simulink model "ASM2d_Influentmodel"  (Simulink 7.0)
settings: Solver=ode45  StartTime=0.0  StopTime=728.0  RelTol=1e-6
values from neighbouring files (symbols this model uses):
  aHpercent = 75    [ASM2d_Influent_init.m]    (also in ASM3_Influent_init.m)
  CODpart_gperPEperd = 115.08    [ASM2d_Influent_init.m]    (also in ASM3_Influent_init.m)
  CODpart_HH_max = 20*CODpart_gperPEperd*PE    (= 184128)    [ASM2d_Influent_init.m]    (also in ASM3_Influent_init.m)
  CODpart_HH_min = 0.1    [ASM2d_Influent_init.m]    (also in ASM3_Influent_init.m)
  CODpart_HH_ns = 35000    [ASM2d_Influent_init.m]    (also in ASM3_Influent_init.m)
  CODpart_HH_nv = factor1*CODpart_gperPEperd*PE    (= 18412.8)    [ASM2d_Influent_init.m]    (also in ASM3_Influent_init.m)
  CODpart_HH_st = 1/24    (= 0.0416666666667)    [ASM2d_Influent_init.m]    (also in ASM3_Influent_init.m)
  CODpart_Ind_kgperd = 2301.80    (= 2301.8)    [ASM2d_Influent_init.m]    (also in ASM3_Influent_init.m)
  CODpart_Ind_max = 20*CODpart_Ind_kgperd    (= 46036)    [ASM2d_Influent_init.m]    (also in ASM3_Influent_init.m)
  CODpart_Ind_min = 0.1    [ASM2d_Influent_init.m]    (also in ASM3_Influent_init.m)
  CODpart_Ind_ns = 21000    [ASM2d_Influent_init.m]    (also in ASM3_Influent_init.m)
  CODpart_Ind_nv = factor2*CODpart_Ind_kgperd    (= 4603.6)    [ASM2d_Influent_init.m]    (also in ASM3_Influent_init.m)
  CODpart_Ind_st = 1/24    (= 0.0416666666667)    [ASM2d_Influent_init.m]    (also in ASM3_Influent_init.m)
  CODsol_gperPEperd = 19.31    [ASM2d_Influent_init.m]    (also in ASM3_Influent_init.m)
  CODsol_HH_max = 20*CODsol_gperPEperd*PE    (= 30896)    [ASM2d_Influent_init.m]    (also in ASM3_Influent_init.m)
  CODsol_HH_min = 0.1    [ASM2d_Influent_init.m]    (also in ASM3_Influent_init.m)
  CODsol_HH_ns = 25000    [ASM2d_Influent_init.m]    (also in ASM3_Influent_init.m)
  CODsol_HH_nv = factor1*2*CODsol_gperPEperd*PE    (= 6179.2)    [ASM2d_Influent_init.m]    (also in ASM3_Influent_init.m)
  CODsol_HH_st = 1/24    (= 0.0416666666667)    [ASM2d_Influent_init.m]    (also in ASM3_Influent_init.m)
  CODsol_Ind_kgperd = 386.24    [ASM2d_Influent_init.m]    (also in ASM3_Influent_init.m)
  CODsol_Ind_max = 20*CODsol_Ind_kgperd    (= 7724.8)    [ASM2d_Influent_init.m]    (also in ASM3_Influent_init.m)
  CODsol_Ind_min = 0.1    [ASM2d_Influent_init.m]    (also in ASM3_Influent_init.m)
  CODsol_Ind_ns = 11000    [ASM2d_Influent_init.m]    (also in ASM3_Influent_init.m)
  CODsol_Ind_nv = factor2*CODsol_Ind_kgperd    (= 772.48)    [ASM2d_Influent_init.m]    (also in ASM3_Influent_init.m)
  CODsol_Ind_st = 1/24    (= 0.0416666666667)    [ASM2d_Influent_init.m]    (also in ASM3_Influent_init.m)
  FFfraction = 0.25    [ASM2d_Influent_init.m]    (also in ASM3_Influent_init.m)
  HHnoiseswitch = 1    [ASM2d_Influent_init.m]    (also in ASM3_Influent_init.m)
  HHpolnoiseswitch = 1    [ASM2d_Influent_init.m]    (also in ASM3_Influent_init.m)
  HHpopswitch = 100    [ASM2d_Influent_init.m]    (also in ASM3_Influent_init.m)
  Indnoiseswitch = 1    [ASM2d_Influent_init.m]    (also in ASM3_Influent_init.m)
  Indpolnoiseswitch = 1    [ASM2d_Influent_init.m]    (also in ASM3_Influent_init.m)
  Indpopswitch = 100    [ASM2d_Influent_init.m]    (also in ASM3_Influent_init.m)
  InfAmp = 1200    [ASM2d_Influent_init.m]    (also in ASM3_Influent_init.m)
  InfBias = 7100    [ASM2d_Influent_init.m]    (also in ASM3_Influent_init.m)
  Infcst = 7100    [ASM2d_Influent_init.m]    (also in ASM3_Influent_init.m)
  InfFreq = 2*pi/364    (= 0.0172614980966)    [ASM2d_Influent_init.m]    (also in ASM3_Influent_init.m)
  InfPhase = -pi*15/24    (= -1.96349540849)    [ASM2d_Influent_init.m]    (also in ASM3_Influent_init.m)
  iSS_XB = 0.90    (= 0.9)    [ASM2d_Influent_init.m]
  iSS_XI = 0.75    [ASM2d_Influent_init.m]
  iSS_XMe = 1.00    (= 1)    [ASM2d_Influent_init.m]
  iSS_XPHA = 0.60    (= 0.6)    [ASM2d_Influent_init.m]
  iSS_XPP = 3.23    [ASM2d_Influent_init.m]
  iSS_XS = 0.75    [ASM2d_Influent_init.m]
  LLrain = 3.5    [ASM2d_Influent_init.m]    (also in ASM3_Influent_init.m)
  PE = 80    [ASM2d_Influent_init.m]    (also in ASM3_Influent_init.m)
  PO4_gperPEperd = (6.89*0.85)/4    (= 1.464125)    [ASM2d_Influent_init.m]
  PO4_HH_max = 20*PO4_gperPEperd*PE    (= 2342.6)    [ASM2d_Influent_init.m]
  PO4_HH_min = 0.1    [ASM2d_Influent_init.m]
  PO4_HH_ns = 55000    [ASM2d_Influent_init.m]
  PO4_HH_nv = factor1*2*PO4_gperPEperd*PE    (= 468.52)    [ASM2d_Influent_init.m]
  PO4_HH_st = 1/24    (= 0.0416666666667)    [ASM2d_Influent_init.m]
  PO4_Ind_kgperd = (61.25*0.85)/4    (= 13.015625)    [ASM2d_Influent_init.m]
  PO4_Ind_max = 20*PO4_Ind_kgperd    (= 260.3125)    [ASM2d_Influent_init.m]
  PO4_Ind_min = 0.1    [ASM2d_Influent_init.m]
  PO4_Ind_ns = 41000    [ASM2d_Influent_init.m]
  PO4_Ind_nv = factor2*PO4_Ind_kgperd    (= 26.03125)    [ASM2d_Influent_init.m]
  PO4_Ind_st = 1/24    (= 0.0416666666667)    [ASM2d_Influent_init.m]
  polnoiseswitch = 1    [ASM2d_Influent_init.m]    (also in ASM3_Influent_init.m)
  Q_HH_ns = 3857    [ASM2d_Influent_init.m]    (also in ASM3_Influent_init.m)
  Q_HH_nv = 4000    [ASM2d_Influent_init.m]    (also in ASM3_Influent_init.m)
  Q_HH_st = 1/24    (= 0.0416666666667)    [ASM2d_Influent_init.m]    (also in ASM3_Influent_init.m)
  Q_Ind_ns = 2000    [ASM2d_Influent_init.m]    (also in ASM3_Influent_init.m)
  Q_Ind_nv = 15000    [ASM2d_Influent_init.m]    (also in ASM3_Influent_init.m)
  Q_Ind_st = 1/24    (= 0.0416666666667)    [ASM2d_Influent_init.m]    (also in ASM3_Influent_init.m)
  Q_SCI_ns = 1000    [ASM2d_Influent_init.m]    (also in ASM3_Influent_init.m)
  Q_SCI_nv = 0.1*InfBias    (= 710)    [ASM2d_Influent_init.m]    (also in ASM3_Influent_init.m)
  Q_SCI_st = 1    [ASM2d_Influent_init.m]    (also in ASM3_Influent_init.m)
  QHHsatmax = QperPE*50    (= 7500)    [ASM2d_Influent_init.m]    (also in ASM3_Influent_init.m)
  QHHsatmin = 0.001    [ASM2d_Influent_init.m]    (also in ASM3_Influent_init.m)
  QInd_weekday = 2500    [ASM2d_Influent_init.m]    (also in ASM3_Influent_init.m)
  QIndsatmax = QInd_weekday*10    (= 25000)    [ASM2d_Influent_init.m]    (also in ASM3_Influent_init.m)
  QIndsatmin = 0.001    [ASM2d_Influent_init.m]    (also in ASM3_Influent_init.m)
  Qpermm = 1500    [ASM2d_Influent_init.m]    (also in ASM3_Influent_init.m)
  QperPE = 150    [ASM2d_Influent_init.m]    (also in ASM3_Influent_init.m)
  QSCIsatmax = 2*(InfBias+InfAmp)    (= 16600)    [ASM2d_Influent_init.m]    (also in ASM3_Influent_init.m)
  QSCIsatmin = 0.0    (= 0)    [ASM2d_Influent_init.m]    (also in ASM3_Influent_init.m)
  rain_nm = 1    [ASM2d_Influent_init.m]    (also in ASM3_Influent_init.m)
  rain_ns = 3000    [ASM2d_Influent_init.m]    (also in ASM3_Influent_init.m)
  rain_nv = 400    [ASM2d_Influent_init.m]    (also in ASM3_Influent_init.m)
  rain_st = 1/24    (= 0.0416666666667)    [ASM2d_Influent_init.m]    (also in ASM3_Influent_init.m)
  rainmax = 1000    [ASM2d_Influent_init.m]    (also in ASM3_Influent_init.m)
  rainmin = 0    [ASM2d_Influent_init.m]    (also in ASM3_Influent_init.m)
  rainpopswitch = 100    [ASM2d_Influent_init.m]    (also in ASM3_Influent_init.m)
  SA_max = 100*Sa_in    (= 2780)    [ASM2d_Influent_init.m]
  SA_min = 0.1    [ASM2d_Influent_init.m]
  SA_ns = 03122    (= 3122)    [ASM2d_Influent_init.m]
  SA_nv = factor3*(Sa_in)    (= 55.6)    [ASM2d_Influent_init.m]
  SA_st = 1/24    (= 0.0416666666667)    [ASM2d_Influent_init.m]
  SCInoiseswitch = 0    [ASM2d_Influent_init.m]    (also in ASM3_Influent_init.m)
  SCIpopswitch = 100    [ASM2d_Influent_init.m]    (also in ASM3_Influent_init.m)
  SF_max = 100*Sf_in    (= 4170)    [ASM2d_Influent_init.m]
  SF_min = 0.1    [ASM2d_Influent_init.m]
  SF_ns = 23122    [ASM2d_Influent_init.m]
  SF_nv = factor3*(Sf_in)    (= 83.4)    [ASM2d_Influent_init.m]
  SF_st = 1/24    (= 0.0416666666667)    [ASM2d_Influent_init.m]
  SI_max = 100*Si_in    (= 3000)    [ASM2d_Influent_init.m]    (also in ASM3_Influent_init.m)
  SI_min = 0.1    [ASM2d_Influent_init.m]    (also in ASM3_Influent_init.m)
  SI_ns = 13122    [ASM2d_Influent_init.m]    (also in ASM3_Influent_init.m)
  SI_nv = factor3*(Si_in)    (= 60)    [ASM2d_Influent_init.m]    (also in ASM3_Influent_init.m)
  SI_st = 1/24    (= 0.0416666666667)    [ASM2d_Influent_init.m]    (also in ASM3_Influent_init.m)
  SNH_gperPEperd = 6.89*0.85    (= 5.8565)    [ASM2d_Influent_init.m]    (also in ASM3_Influent_init.m)
  SNH_HH_max = 20*SNH_gperPEperd*PE    (= 9370.4)    [ASM2d_Influent_init.m]    (also in ASM3_Influent_init.m)
  SNH_HH_min = 0.1    [ASM2d_Influent_init.m]    (also in ASM3_Influent_init.m)
  SNH_HH_ns = 45000    [ASM2d_Influent_init.m]    (also in ASM3_Influent_init.m)
  SNH_HH_nv = factor1*2*SNH_gperPEperd*PE    (= 1874.08)    [ASM2d_Influent_init.m]    (also in ASM3_Influent_init.m)
  SNH_HH_st = 1/24    (= 0.0416666666667)    [ASM2d_Influent_init.m]    (also in ASM3_Influent_init.m)
  SNH_Ind_kgperd = 61.25*0.85    (= 52.0625)    [ASM2d_Influent_init.m]    (also in ASM3_Influent_init.m)
  SNH_Ind_max = 20*SNH_Ind_kgperd    (= 1041.25)    [ASM2d_Influent_init.m]    (also in ASM3_Influent_init.m)
  SNH_Ind_min = 0.1    [ASM2d_Influent_init.m]    (also in ASM3_Influent_init.m)
  SNH_Ind_ns = 31000    [ASM2d_Influent_init.m]    (also in ASM3_Influent_init.m)
  SNH_Ind_nv = factor2*SNH_Ind_kgperd    (= 104.125)    [ASM2d_Influent_init.m]    (also in ASM3_Influent_init.m)
  SNH_Ind_st = 1/24    (= 0.0416666666667)    [ASM2d_Influent_init.m]    (also in ASM3_Influent_init.m)
  SNH_max = 100*Snh_in    (= 3156)    [ASM2d_Influent_init.m]    (also in ASM3_Influent_init.m)
  SNH_min = 0.1    [ASM2d_Influent_init.m]    (also in ASM3_Influent_init.m)
  SNH_ns = 63122    [ASM2d_Influent_init.m]    (also in ASM3_Influent_init.m)
  SNH_nv = factor3*(Snh_in)    (= 63.12)    [ASM2d_Influent_init.m]    (also in ASM3_Influent_init.m)
  SNH_st = 1/24    (= 0.0416666666667)    [ASM2d_Influent_init.m]    (also in ASM3_Influent_init.m)
  SPO4_ns = 73122    [ASM2d_Influent_init.m]
  SPO4_nv = factor3*(Spo4_in)    (= 18.02)    [ASM2d_Influent_init.m]
  SPO4_st = 1/24    (= 0.0416666666667)    [ASM2d_Influent_init.m]
  ... (+24 more)
libraries: simulink x5
(part 2 of 2)

== system ASM2d_Influentmodel/ASM2d/sewer/sewer4 ==
  In1 : Inport  OutDataType=sfix(16)  OutScaling=2^0
  Constant : Constant  OutDataType=sfix(16)  OutScaling=2^0
  Mux1 : Mux  Inputs=2
  S-Function : S-Function  FunctionName=sewer_asm2d  Parameters=ASM2d_SEWERINIT, ASM2d_PARS, SPAR
  S-Function1 : S-Function  FunctionName=sewer_asm2d  Parameters=ASM2d_SEWERINIT, ASM2d_PARS, SPAR
  S-Function2 : S-Function  FunctionName=sewer_asm2d  Parameters=ASM2d_SEWERINIT, ASM2d_PARS, SPAR
  Selector9 : Selector  InputPortWidth=27  IndexOptions=Index vector (dialog)  Indices=[1 2 3 4 5 6 7 8 9 10 11 12 13 14 15 16 17 18 19 20 21 22 23 24 25 26 ]  OutputSizes=1
  Out1 : Outport
  wires:
  S-Function/1 -> S-Function1/1
  S-Function1/1 -> S-Function2/1
  S-Function2/1 -> Selector9/1
  Mux1/1 -> S-Function/1
  Constant/1 -> Mux1/2
  In1/1 -> Mux1/1
  Selector9/1 -> Out1/1

== system ASM2d_Influentmodel/ASM2d/sewer/sewer5 ==
  In1 : Inport  OutDataType=sfix(16)  OutScaling=2^0
  Constant : Constant  OutDataType=sfix(16)  OutScaling=2^0
  Mux1 : Mux  Inputs=2
  S-Function : S-Function  FunctionName=sewer_asm2d  Parameters=ASM2d_SEWERINIT, ASM2d_PARS, SPAR
  S-Function1 : S-Function  FunctionName=sewer_asm2d  Parameters=ASM2d_SEWERINIT, ASM2d_PARS, SPAR
  S-Function2 : S-Function  FunctionName=sewer_asm2d  Parameters=ASM2d_SEWERINIT, ASM2d_PARS, SPAR
  Selector9 : Selector  InputPortWidth=27  IndexOptions=Index vector (dialog)  Indices=[1 2 3 4 5 6 7 8 9 10 11 12 13 14 15 16 17 18 19 20 21 22 23 24 25 26 ]  OutputSizes=1
  Out1 : Outport
  wires:
  S-Function/1 -> S-Function1/1
  S-Function1/1 -> S-Function2/1
  S-Function2/1 -> Selector9/1
  Mux1/1 -> S-Function/1
  Constant/1 -> Mux1/2
  In1/1 -> Mux1/1
  Selector9/1 -> Out1/1

== system ASM2d_Influentmodel/ASM2d/sewer/sewer6 ==
  In1 : Inport  OutDataType=sfix(16)  OutScaling=2^0
  Constant : Constant  OutDataType=sfix(16)  OutScaling=2^0
  Mux1 : Mux  Inputs=2
  S-Function : S-Function  FunctionName=sewer_asm2d  Parameters=ASM2d_SEWERINIT, ASM2d_PARS, SPAR
  S-Function1 : S-Function  FunctionName=sewer_asm2d  Parameters=ASM2d_SEWERINIT, ASM2d_PARS, SPAR
  S-Function2 : S-Function  FunctionName=sewer_asm2d  Parameters=ASM2d_SEWERINIT, ASM2d_PARS, SPAR
  Selector9 : Selector  InputPortWidth=27  IndexOptions=Index vector (dialog)  Indices=[1 2 3 4 5 6 7 8 9 10 11 12 13 14 15 16 17 18 19 20 21 22 23 24 25 26 ]  OutputSizes=1
  Out1 : Outport
  wires:
  S-Function/1 -> S-Function1/1
  S-Function1/1 -> S-Function2/1
  S-Function2/1 -> Selector9/1
  Mux1/1 -> S-Function/1
  Constant/1 -> Mux1/2
  In1/1 -> Mux1/1
  Selector9/1 -> Out1/1

== system ASM2d_Influentmodel/ASM2d/sewer/sewer7 ==
  In1 : Inport  OutDataType=sfix(16)  OutScaling=2^0
  Constant : Constant  OutDataType=sfix(16)  OutScaling=2^0
  Mux1 : Mux  Inputs=2
  S-Function : S-Function  FunctionName=sewer_asm2d  Parameters=ASM2d_SEWERINIT, ASM2d_PARS, SPAR
  S-Function1 : S-Function  FunctionName=sewer_asm2d  Parameters=ASM2d_SEWERINIT, ASM2d_PARS, SPAR
  S-Function2 : S-Function  FunctionName=sewer_asm2d  Parameters=ASM2d_SEWERINIT, ASM2d_PARS, SPAR
  Selector9 : Selector  InputPortWidth=27  IndexOptions=Index vector (dialog)  Indices=[1 2 3 4 5 6 7 8 9 10 11 12 13 14 15 16 17 18 19 20 21 22 23 24 25 26 ]  OutputSizes=1
  Out1 : Outport
  wires:
  S-Function/1 -> S-Function1/1
  S-Function1/1 -> S-Function2/1
  S-Function2/1 -> Selector9/1
  Mux1/1 -> S-Function/1
  Constant/1 -> Mux1/2
  In1/1 -> Mux1/1
  Selector9/1 -> Out1/1

== system ASM2d_Influentmodel/ASM2d/sewer/sewer8 ==
  In1 : Inport  OutDataType=sfix(16)  OutScaling=2^0
  Constant : Constant  OutDataType=sfix(16)  OutScaling=2^0
  Mux1 : Mux  Inputs=2
  S-Function : S-Function  FunctionName=sewer_asm2d  Parameters=ASM2d_SEWERINIT, ASM2d_PARS, SPAR
  S-Function1 : S-Function  FunctionName=sewer_asm2d  Parameters=ASM2d_SEWERINIT, ASM2d_PARS, SPAR
  S-Function2 : S-Function  FunctionName=sewer_asm2d  Parameters=ASM2d_SEWERINIT, ASM2d_PARS, SPAR
  Selector9 : Selector  InputPortWidth=27  IndexOptions=Index vector (dialog)  Indices=[1 2 3 4 5 6 7 8 9 10 11 12 13 14 15 16 17 18 19 20 21 22 23 24 25 26 ]  OutputSizes=1
  Out1 : Outport
  wires:
  S-Function/1 -> S-Function1/1
  S-Function1/1 -> S-Function2/1
  S-Function2/1 -> Selector9/1
  Mux1/1 -> S-Function/1
  Constant/1 -> Mux1/2
  In1/1 -> Mux1/1
  Selector9/1 -> Out1/1
